simulink model "AME552_HW2_P2_SimulinkModel"  (R2024b)
settings: Solver=VariableStepAuto  StartTime=0.0  StopTime=5  RelTol=1e-3
values from neighbouring files (symbols this model uses):
  alpha = 1    [AME552_HW2_P2.m]    (also in AME552_HW2_P2_Simulink.m)
  beta = 1    [AME552_HW2_P2.m]    (also in AME552_HW2_P2_Simulink.m)
  D = 1    [AME552_HW2_P2.m]    (also in AME552_HW2_P2_Simulink.m)
  de0 = de0_space(j)    [AME552_HW2_P2_Simulink.m]
  e0 = e0_space(i)    [AME552_HW2_P2_Simulink.m]
  M = 1    [AME552_HW2_P2.m]    (also in AME552_HW2_P2_Simulink.m)
libraries: simulink x1
settings Model: Creator=lewis  LastModifiedBy=lewis

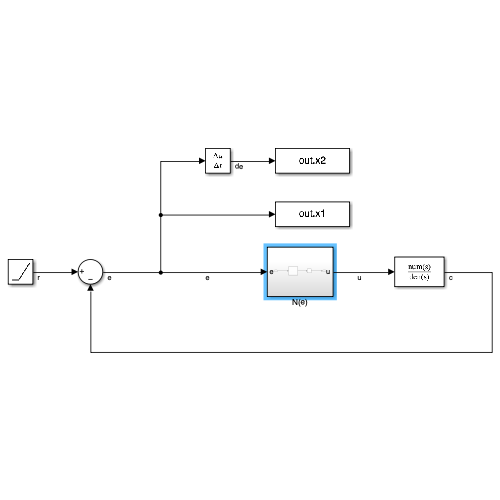
[thumbnail: Simulink's stored preview of the top-level diagram]
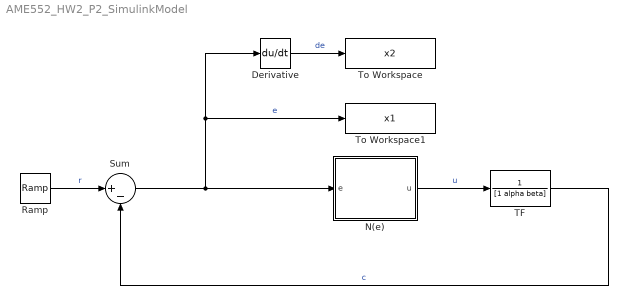
== system AME552_HW2_P2_SimulinkModel ==
  Derivative : Derivative
  N(e) : Subsystem
  Ramp : simulink/Sources/Ramp  slope=de0  start=0  InitialOutput=e0
  Sum : Sum  Inputs=|+-
  TF : TransferFcn  Denominator=[1 alpha beta]
  To Workspace : ToWorkspace  VariableName=x2  SaveFormat=Timeseries  SampleTime=-1
  To Workspace1 : ToWorkspace  VariableName=x1  SaveFormat=Timeseries  SampleTime=-1
  wires:
  Sum/1 -> N(e)/1(e), To Workspace1/1, Derivative/1  "e"
  TF/1 -> Sum/2  "c"
  Derivative/1 -> To Workspace/1  "de"
  N(e)/1(u) -> TF/1  "u"
  Ramp/1 -> Sum/1  "r"

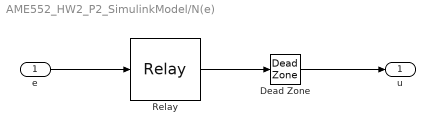
== system AME552_HW2_P2_SimulinkModel/N(e) ==
  e : Inport
  Dead Zone : DeadZone  LowerValue=-D  UpperValue=D
  Relay : Relay  OnSwitchValue=D  OffSwitchValue=-D  OnOutputValue=M+D  OffOutputValue=-M-D
  u : Outport
  wires:
  e/1 -> Relay/1
  Dead Zone/1 -> u/1
  Relay/1 -> Dead Zone/1
